simulink model "PID_digital_tarea"  (R2016b)
settings: Solver=ode45  StartTime=0.0  StopTime=10  MaxStep=1e-5  RelTol=1e-3  EnableMultiTasking=on
values from neighbouring files (symbols this model uses):
  T = 0.15    [tp2.m]
undefined symbols (not defined in the file or in its folder): DiscIntNeverNeededParam
libraries: simulink x1
settings Model: Creator=Usuario  LastModifiedBy=Mauricio
settings DataIOCC: SaveFormat=Array  SignalLoggingSaveFormat=ModelDataLogs
settings OptimizationCC: InitFltsAndDblsToZero=on  LifeSpan=inf
settings DebuggingCC: SaveWithParameterizedLinksMsg=none  UnderspecifiedInitializationDetection=Classic  MergeDetectMultiDrivingBlocksExec=none  SignalResolutionControl=TryResolveAllWithWarning  SolverPrmCheckMsg=warning  MultiTaskDSMMsg=warning  MultiTaskCondExecSysMsg=none  FcnCallInpInsideContextMsg=warning  SFUnexpectedBacktrackingDiag=warning  SFNoUnconditionalDefaultTransitionDiag=warning  SFExecutionAtInitializationDiag=none
settings HardwareCC: ProdBitPerPointer=32  ProdBitPerSizeT=32  ProdBitPerPtrDiffT=32  ProdLargestAtomicFloat=None  ProdIntDivRoundTo=Undefined  ProdEndianess=Unspecified  ProdWordSize=32  ProdHWDeviceType=32-bit Generic
settings ModelReferenceCC: PropagateSignalLabelsOutOfModel=off
settings GRTTargetCC: TargetFcnLib=ansi_tfl_tmw.mat  TargetLangStandard=C89/C90 (ANSI)  GeneratePreprocessorConditionals=Disable all  CombineOutputUpdateFcns=off  GRTInterface=on
settings ConfigComp: CovMetricSettings=dw  CovHtmlReporting=on  CovSaveCumulativeToWorkspaceVar=on  CovSaveSingleToWorkspaceVar=on  CovExternalEMLEnable=off  CovSFcnEnable=off

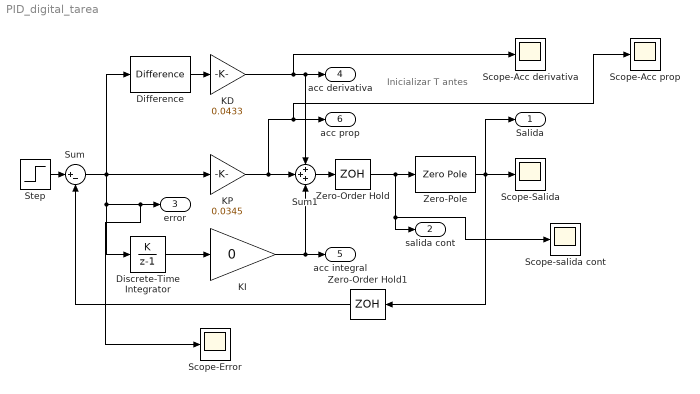
== system PID_digital_tarea ==
  note: Inicializar T antes
  Difference : simulink/Discrete/Difference  ICPrevInput=0.0  InputProcessing=Inherited  OutMin=[]  OutMax=[]  OutDataType=fixdt(1, 16)  OutScaling=2^-10  DoSatur=off
  Discrete-Time Integrator : DiscreteIntegrator  IntegratorMethod=Accumulation: Forward Euler  SampleTime=-1  ICPrevOutput=DiscIntNeverNeededParam  ICPrevScaledInput=DiscIntNeverNeededParam
  KD : Gain  Gain=0.0433
  KI : Gain  Gain=0
  KP : Gain  Gain=0.0345
  Scope-Acc derivativa : Scope
  Scope-Acc prop : Scope
  Scope-Error : Scope
  Scope-Salida : Scope
  Scope-salida cont : Scope
  Step : Step  Time=0  SampleTime=T
  Sum : Sum  Inputs=|+-
  Sum1 : Sum  Inputs=+++
  Zero-Order Hold : ZeroOrderHold  SampleTime=T
  Zero-Order Hold1 : ZeroOrderHold  SampleTime=T
  Zero-Pole : ZeroPole  Zeros=[-10]  Poles=[0 -2]  Gain=[10]
  Salida : Outport
  salida cont : Outport  Port=2
  error : Outport  Port=3
  acc derivativa : Outport  Port=4
  acc integral : Outport  Port=5
  acc prop : Outport  Port=6
  wires:
  Zero-Order Hold/1 -> Zero-Pole/1, Scope-salida cont/1, salida cont/1
  Step/1 -> Sum/1
  Zero-Pole/1 -> Zero-Order Hold1/1, Scope-Salida/1, Salida/1
  KI/1 -> Sum1/3, acc integral/1
  KP/1 -> Scope-Acc prop/1, acc prop/1, Sum1/2
  Zero-Order Hold1/1 -> Sum/2
  Sum/1 -> Difference/1, Discrete-Time Integrator/1, Scope-Error/1, error/1, KP/1
  Sum1/1 -> Zero-Order Hold/1
  KD/1 -> Scope-Acc derivativa/1, Sum1/1, acc derivativa/1
  Difference/1 -> KD/1
  Discrete-Time Integrator/1 -> KI/1
